simulink model "gm_RNN_MAC"  (R2020b)
settings: Solver=VariableStepAuto  StartTime=0.0  StopTime=10.0  RelTol=1e-3
libraries: hdlmdlgenlib x2
settings Model: Creator=chank  LastModifiedBy=chank
settings OptimizationCC: BlockReduction=off  ConditionallyExecuteInputs=off
settings DebuggingCC: InheritedTsInSrcMsg=none

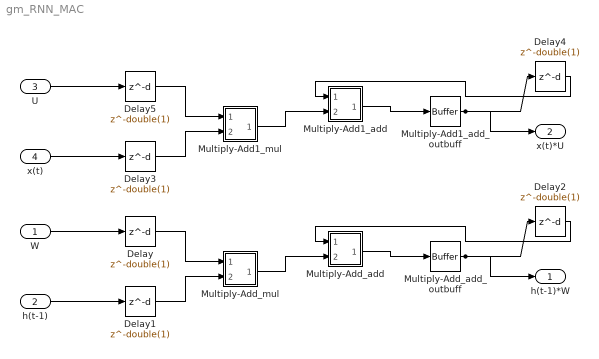
== system gm_RNN_MAC ==
  W : Inport  OutDataTypeStr=single  PortDimensions=1  SampleTime=0.2
  h(t-1) : Inport  Port=2  OutDataTypeStr=single  PortDimensions=1  SampleTime=0.2
  U : Inport  Port=3  OutDataTypeStr=single  PortDimensions=1  SampleTime=0.2
  x(t) : Inport  Port=4  OutDataTypeStr=single  PortDimensions=1  SampleTime=0.2
  Delay{,1..5} (6 alike) : Delay  DelayLength=double(1)  InitialCondition=0  SampleTime=0.2
  Multiply-Add1_add : Subsystem
      mask Display: disp('NFP\nadd');
  Multiply-Add1_add_outbuff : hdlmdlgenlib/Buffer
      settings: SourceProductBaseCode=SL
  Multiply-Add1_mul : Subsystem
      mask Display: disp('NFP\nmul');
  Multiply-Add_add : Subsystem
      mask Display: disp('NFP\nadd');
  Multiply-Add_add_outbuff : hdlmdlgenlib/Buffer
      settings: SourceProductBaseCode=SL
  Multiply-Add_mul : Subsystem
      mask Display: disp('NFP\nmul');
  h(t-1)*W : Outport
  x(t)*U : Outport  Port=2
  wires:
  W/1 -> Delay/1
  h(t-1)/1 -> Delay1/1
  U/1 -> Delay5/1
  x(t)/1 -> Delay3/1
  Delay/1 -> Multiply-Add_mul/1(In1)
  Delay1/1 -> Multiply-Add_mul/2(In2)
  Delay2/1 -> Multiply-Add_add/1(In1)
  Delay3/1 -> Multiply-Add1_mul/2(In2)
  Delay4/1 -> Multiply-Add1_add/1(In1)
  Delay5/1 -> Multiply-Add1_mul/1(In1)
  Multiply-Add_add_outbuff/1 -> Delay2/1, h(t-1)*W/1
  Multiply-Add1_add_outbuff/1 -> Delay4/1, x(t)*U/1
  Multiply-Add_mul/1(Out1) -> Multiply-Add_add/2(In2)
  Multiply-Add_add/1(Out1) -> Multiply-Add_add_outbuff/1
  Multiply-Add1_mul/1(Out1) -> Multiply-Add1_add/2(In2)
  Multiply-Add1_add/1(Out1) -> Multiply-Add1_add_outbuff/1

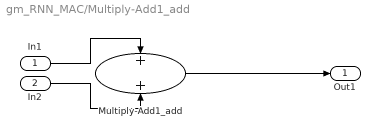
== system gm_RNN_MAC/Multiply-Add1_add ==
  In1 : Inport
  In2 : Inport  Port=2
  Multiply-Add1_add : Sum  OutDataTypeStr=single  SampleTime=0.2
  Out1 : Outport
  wires:
  In1/1 -> Multiply-Add1_add/1
  In2/1 -> Multiply-Add1_add/2
  Multiply-Add1_add/1 -> Out1/1

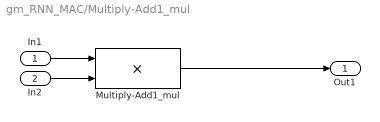
== system gm_RNN_MAC/Multiply-Add1_mul ==
  In1 : Inport
  In2 : Inport  Port=2
  Multiply-Add1_mul : Product  Inputs=**  OutDataTypeStr=single  SampleTime=0.2
  Out1 : Outport
  wires:
  In1/1 -> Multiply-Add1_mul/1
  In2/1 -> Multiply-Add1_mul/2
  Multiply-Add1_mul/1 -> Out1/1

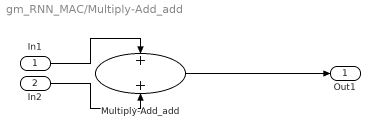
== system gm_RNN_MAC/Multiply-Add_add ==
  In1 : Inport
  In2 : Inport  Port=2
  Multiply-Add_add : Sum  OutDataTypeStr=single  SampleTime=0.2
  Out1 : Outport
  wires:
  In1/1 -> Multiply-Add_add/1
  In2/1 -> Multiply-Add_add/2
  Multiply-Add_add/1 -> Out1/1

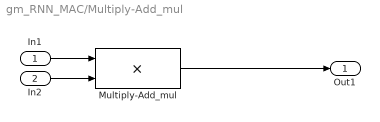
== system gm_RNN_MAC/Multiply-Add_mul ==
  In1 : Inport
  In2 : Inport  Port=2
  Multiply-Add_mul : Product  Inputs=**  OutDataTypeStr=single  SampleTime=0.2
  Out1 : Outport
  wires:
  In1/1 -> Multiply-Add_mul/1
  In2/1 -> Multiply-Add_mul/2
  Multiply-Add_mul/1 -> Out1/1
